simulink model "Controller_CS3"  (R2014a)
settings: Solver=ode4  StartTime=0.0  StopTime=Inf  FixedStep=0.01  MaxStep=0.01  RelTol=1e-3
undefined symbols (not defined in the file): Control, T_m_inv, T_matrix
libraries: simulink_extras x4, commnoisgen2 x1
(part 2 of 3)

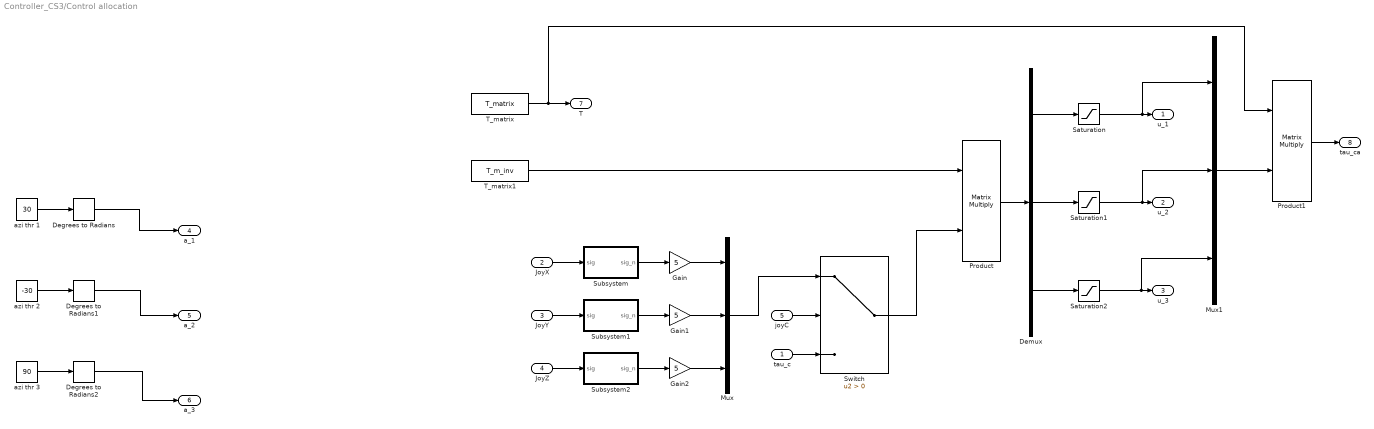
== system Controller_CS3/Control allocation ==
  tau_c : Inport  PortDimensions=3
  JoyX : Inport  Port=2  PortDimensions=1
  JoyY : Inport  Port=3  PortDimensions=1
  JoyZ : Inport  Port=4  PortDimensions=1
  joyC : Inport  Port=5  PortDimensions=1
  Degrees to Radians : simulink_extras/Transformations/Degrees to Radians
  Degrees to Radians1 : simulink_extras/Transformations/Degrees to Radians
  Degrees to Radians2 : simulink_extras/Transformations/Degrees to Radians
  Demux : Demux  Outputs=3
  Gain : Gain  Gain=5
  Gain1 : Gain  Gain=5
  Gain2 : Gain  Gain=5
  Mux : Mux  Inputs=3
  Mux1 : Mux  Inputs=3
  Product : Product  Multiplication=Matrix(*)
  Product1 : Product  Multiplication=Matrix(*)
  Saturation : Saturate  UpperLimit=13  LowerLimit=-13
  Saturation1 : Saturate  UpperLimit=13  LowerLimit=-13
  Saturation2 : Saturate  UpperLimit=8  LowerLimit=-8
  Subsystem : Subsystem
  Subsystem1 : Subsystem
  Subsystem2 : Subsystem
  Switch : Switch  Criteria=u2 > Threshold
  T_matrix : Constant  Value=T_matrix  VectorParams1D=off
  T_matrix1 : Constant  Value=T_m_inv  VectorParams1D=off
  azi thr 1 : Constant  Value=30
  azi thr 2 : Constant  Value=-30
  azi thr 3 : Constant  Value=90
  u_1 : Outport  PortDimensions=1
  u_2 : Outport  Port=2  PortDimensions=1
  u_3 : Outport  Port=3  PortDimensions=1
  a_1 : Outport  Port=4
  a_2 : Outport  Port=5
  a_3 : Outport  Port=6
  T : Outport  Port=7
  tau_ca : Outport  Port=8
  wires:
  azi thr 1/1 -> Degrees to Radians/1
  azi thr 2/1 -> Degrees to Radians1/1
  azi thr 3/1 -> Degrees to Radians2/1
  Degrees to Radians/1 -> a_1/1
  Degrees to Radians1/1 -> a_2/1
  Degrees to Radians2/1 -> a_3/1
  Product/1 -> Demux/1
  T_matrix1/1 -> Product/1
  JoyX/1 -> Subsystem/1(sig)
  JoyY/1 -> Subsystem1/1(sig)
  JoyZ/1 -> Subsystem2/1(sig)
  joyC/1 -> Switch/2
  Subsystem2/1(sig_n) -> Gain2/1
  Subsystem1/1(sig_n) -> Gain1/1
  Subsystem/1(sig_n) -> Gain/1
  Mux/1 -> Switch/1
  tau_c/1 -> Switch/3
  Switch/1 -> Product/2
  Gain/1 -> Mux/1
  Gain1/1 -> Mux/2
  Gain2/1 -> Mux/3
  Mux1/1 -> Product1/2
  T_matrix/1 -> Product1/1, T/1
  Product1/1 -> tau_ca/1
  Demux/3 -> Saturation2/1
  Demux/2 -> Saturation1/1
  Demux/1 -> Saturation/1
  Saturation1/1 -> Mux1/2, u_2/1
  Saturation2/1 -> Mux1/3, u_3/1
  Saturation/1 -> Mux1/1, u_1/1

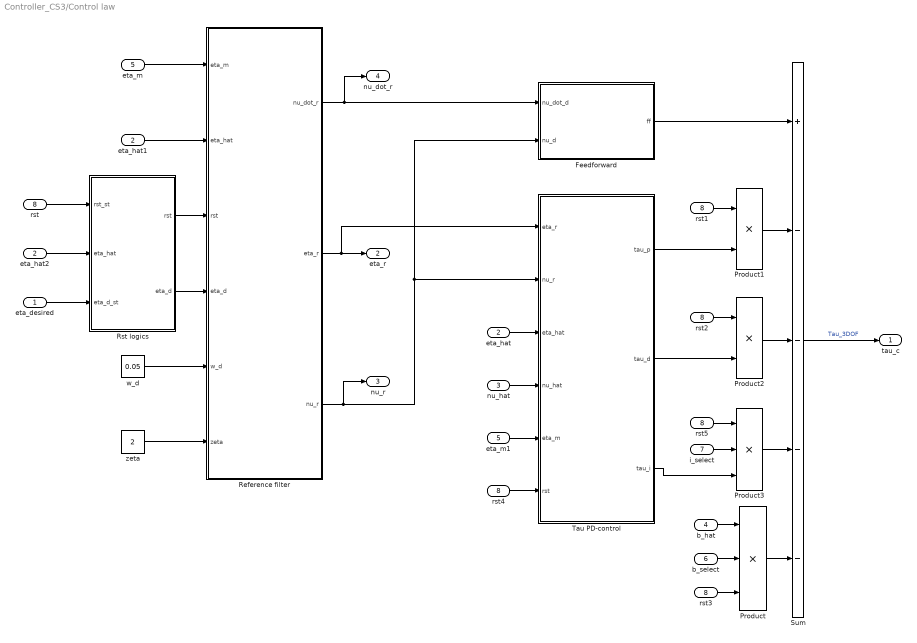
== system Controller_CS3/Control law ==
  eta_desired : Inport
  eta_hat : Inport  Port=2
  nu_hat : Inport  Port=3
  b_hat : Inport  Port=4
  eta_m : Inport  Port=5
  b_select : Inport  Port=6
  i_select : Inport  Port=7
  rst : Inport  Port=8
  Feedforward : Subsystem
  Product : Product  Inputs=3
  Product1 : Product
  Product2 : Product
  Product3 : Product  Inputs=3
  Reference filter : Subsystem
  Rst logics : Subsystem
  Sum : Sum  Inputs=+----  SaturateOnIntegerOverflow=on
  Tau PD-control : Subsystem
  eta_hat1 : InportShadow  Port=2
  eta_hat2 : InportShadow  Port=2
  eta_m1 : InportShadow  Port=5
  rst{1..5} (5 alike) : InportShadow  Port=8
  w_d : Constant  Value=0.05
  zeta : Constant  Value=2
  tau_c : Outport
  eta_r : Outport  Port=2
  nu_r : Outport  Port=3
  nu_dot_r : Outport  Port=4
  wires:
  Sum/1 -> tau_c/1  "Tau_3DOF"
  eta_hat/1 -> Tau PD-control/3(eta_hat)
  nu_hat/1 -> Tau PD-control/4(nu_hat)
  b_hat/1 -> Product/1
  Reference filter/1(nu_dot_r) -> nu_dot_r/1, Feedforward/1(nu_dot_d)
  Reference filter/2(eta_r) -> eta_r/1, Tau PD-control/1(eta_r)
  Reference filter/3(nu_r) -> Feedforward/2(nu_d), Tau PD-control/2(nu_r), nu_r/1
  eta_m1/1 -> Tau PD-control/5(eta_m)
  b_select/1 -> Product/2
  Rst logics/1(rst) -> Reference filter/3(rst)
  Rst logics/2(eta_d) -> Reference filter/4(eta_d)
  eta_m/1 -> Reference filter/1(eta_m)
  eta_desired/1 -> Rst logics/3(eta_d_st)
  rst/1 -> Rst logics/1(rst_st)
  eta_hat1/1 -> Reference filter/2(eta_hat)
  w_d/1 -> Reference filter/5(w_d)
  zeta/1 -> Reference filter/6(zeta)
  Product1/1 -> Sum/2
  rst1/1 -> Product1/1
  rst2/1 -> Product2/1
  rst3/1 -> Product/3
  eta_hat2/1 -> Rst logics/2(eta_hat)
  rst4/1 -> Tau PD-control/6(rst)
  Product/1 -> Sum/5
  Tau PD-control/3(tau_i) -> Product3/3
  rst5/1 -> Product3/1
  Feedforward/1(ff) -> Sum/1
  Product3/1 -> Sum/4
  Product2/1 -> Sum/3
  Tau PD-control/2(tau_d) -> Product2/2
  Tau PD-control/1(tau_p) -> Product1/2
  i_select/1 -> Product3/2

== system Controller_CS3/CyberShip3Model ==
  note: nu
  note: nu_dot
  note: etadot
  tau : Inport
  D : Gain  Gain=Control.VessObs.D  Multiplication=Matrix(K*u)  SaturateOnIntegerOverflow=on  OutDataTypeStr=Inherit: Same as input  ParamDataTypeStr=Inherit: Same as input
  Integrator1 : Integrator
  Integrator2 : Integrator
  Rotation matrix in yaw 1 : Subsystem  AncestorBlock=marine_gnc/Models/ Kinematics/Rotation matrix in yaw
      mask help:
      | b = R(psi)* a
      |
      | where
      |
      | input 1:    psi
      | input 2:    a - vector dim 3
      | output 1:  b - vector dim 3
      mask Display:
      | port_label('output', 1, 'R(psi)*v')
      | port_label('input', 1, 'psi')
      | port_label('input', 2, 'v')
  Sum3 : Sum  Inputs=+-  SaturateOnIntegerOverflow=on  InputSameDT=on  OutDataTypeStr=Inherit: Same as first input
  inv(M) : Gain  Gain=Control.VessObs.M_inv  Multiplication=Matrix(K*u)  SaturateOnIntegerOverflow=on  OutDataTypeStr=Inherit: Same as input  ParamDataTypeStr=Inherit: Same as input
  psi : Selector  InputPortWidth=3  Indices=[3]
  eta : Outport
  nu : Outport  Port=2
  wires:
  Integrator2/1 -> Rotation matrix in yaw 1/2(nu), nu/1, D/1
  D/1 -> Sum3/2
  Sum3/1 -> inv(M)/1
  inv(M)/1 -> Integrator2/1
  Rotation matrix in yaw 1/1(R*nu) -> Integrator1/1
  Integrator1/1 -> eta/1, psi/1
  psi/1 -> Rotation matrix in yaw 1/1(psi)
  tau/1 -> Sum3/1

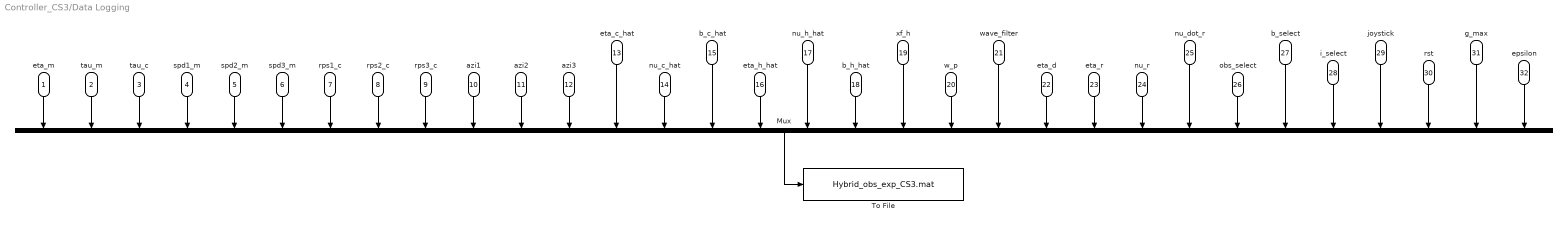
== system Controller_CS3/Data Logging ==
  eta_m : Inport
  tau_m : Inport  Port=2
  tau_c : Inport  Port=3
  spd1_m : Inport  Port=4
  spd2_m : Inport  Port=5
  spd3_m : Inport  Port=6
  rps1_c : Inport  Port=7
  rps2_c : Inport  Port=8
  rps3_c : Inport  Port=9
  azi1 : Inport  Port=10
  azi2 : Inport  Port=11
  azi3 : Inport  Port=12
  eta_c_hat : Inport  Port=13
  nu_c_hat : Inport  Port=14
  b_c_hat : Inport  Port=15
  eta_h_hat : Inport  Port=16
  nu_h_hat : Inport  Port=17
  b_h_hat : Inport  Port=18
  xf_h : Inport  Port=19
  w_p : Inport  Port=20
  wave_filter : Inport  Port=21
  eta_d : Inport  Port=22
  eta_r : Inport  Port=23
  nu_r : Inport  Port=24
  nu_dot_r : Inport  Port=25
  obs_select : Inport  Port=26
  b_select : Inport  Port=27
  i_select : Inport  Port=28
  joystick : Inport  Port=29
  rst : Inport  Port=30
  g_max : Inport  Port=31
  epsilon : Inport  Port=32
  Mux : Mux  Inputs=32
  To File : ToFile  Filename=Hybrid_obs_exp_CS3.mat  MatrixName=data  SampleTime=0.01
  wires:
  eta_m/1 -> Mux/1
  Mux/1 -> To File/1
  tau_m/1 -> Mux/2
  tau_c/1 -> Mux/3
  spd1_m/1 -> Mux/4
  spd2_m/1 -> Mux/5
  spd3_m/1 -> Mux/6
  rps1_c/1 -> Mux/7
  rps2_c/1 -> Mux/8
  rps3_c/1 -> Mux/9
  azi1/1 -> Mux/10
  azi2/1 -> Mux/11
  azi3/1 -> Mux/12
  eta_c_hat/1 -> Mux/13
  nu_c_hat/1 -> Mux/14
  b_c_hat/1 -> Mux/15
  eta_h_hat/1 -> Mux/16
  nu_h_hat/1 -> Mux/17
  b_h_hat/1 -> Mux/18
  xf_h/1 -> Mux/19
  w_p/1 -> Mux/20
  wave_filter/1 -> Mux/21
  eta_r/1 -> Mux/23
  eta_d/1 -> Mux/22
  nu_r/1 -> Mux/24
  obs_select/1 -> Mux/26
  nu_dot_r/1 -> Mux/25
  b_select/1 -> Mux/27
  i_select/1 -> Mux/28
  joystick/1 -> Mux/29
  rst/1 -> Mux/30
  g_max/1 -> Mux/31
  epsilon/1 -> Mux/32

== system Controller_CS3/Fake signal generator ==
  Gain : Gain  Gain=0.5
  Gain1 : Gain  Gain=diag([1 1 0.1])  Multiplication=Matrix(K*u)
  Gain2 : Gain  Gain=0
  Gaussian Noise Generator : commnoisgen2/Gaussian Noise Generator  m=[0 0 0]'  d=[1 1 0.25]'  s=[41 42 45]'  Ts=0.01  frameBased=off  sampPerFrame=1  orient=off  outDataType=double
  Integrator : Integrator
  Integrator1 : Integrator
  Integrator2 : Integrator
  Mux : Mux  Inputs=3
  Step : Step  Time=20  SampleTime=0
  Step1 : Step  Time=30  SampleTime=0
  Step2 : Step  Time=30  After=25*pi/180  SampleTime=0
  Sum : Sum  Inputs=|+-
  Sum1 : Sum  Inputs=|++
  Sum2 : Sum  Inputs=|+-
  eta_f : Outport
  wires:
  Gaussian Noise Generator/1 -> Integrator1/1
  Sum/1 -> Gain/1
  Gain/1 -> Integrator/1
  Integrator1/1 -> Sum/1
  Integrator/1 -> Sum1/1, Sum/2
  Sum1/1 -> Gain1/1
  Step/1 -> Mux/1
  Step1/1 -> Mux/2
  Step2/1 -> Mux/3
  Sum2/1 -> Gain2/1
  Integrator2/1 -> Sum1/2, Sum2/2
  Gain2/1 -> Integrator2/1
  Mux/1 -> Sum2/1
  Gain1/1 -> eta_f/1

== system Controller_CS3/Generalized force computation ==
  rps1 : Inport  PortDimensions=1
  rps2 : Inport  Port=2  PortDimensions=1
  rps3 : Inport  Port=3  PortDimensions=1
  T : Inport  Port=4
  Constant : Constant  Value=0.3507
  Constant1 : Constant  Value=0.2423
  Constant10 : Constant  Value=0.05
  Constant11 : Constant  Value=1024
  Constant2 : Constant  Value=0.09
  Constant3 : Constant  Value=1024
  Constant4 : Constant  Value=0.3464
  Constant5 : Constant  Value=0.2402
  Constant6 : Constant  Value=0.09
  Constant7 : Constant  Value=1024
  Constant8 : Constant  Value=0.1790
  Constant9 : Constant  Value=0.2383
  MATLAB Function : MATLAB Function  TreatAsAtomicUnit=on
  MATLAB Function1 : MATLAB Function  TreatAsAtomicUnit=on
  MATLAB Function2 : MATLAB Function  TreatAsAtomicUnit=on
  Mux : Mux  Inputs=3
  Product : Product  Multiplication=Matrix(*)
  tau_m : Outport
  wires:
  rps2/1 -> MATLAB Function1/1(rps)
  rps3/1 -> MATLAB Function2/1(rps)
  Mux/1 -> Product/2
  Product/1 -> tau_m/1
  T/1 -> Product/1
  Constant/1 -> MATLAB Function/2(Kt_p)
  Constant1/1 -> MATLAB Function/3(Kt_n)
  Constant2/1 -> MATLAB Function/4(d)
  Constant3/1 -> MATLAB Function/5(rho)
  rps1/1 -> MATLAB Function/1(rps)
  MATLAB Function/1(u) -> Mux/1
  Constant4/1 -> MATLAB Function1/2(Kt_p)
  Constant5/1 -> MATLAB Function1/3(Kt_n)
  Constant6/1 -> MATLAB Function1/4(d)
  Constant7/1 -> MATLAB Function1/5(rho)
  Constant8/1 -> MATLAB Function2/3(Kt_n)
  Constant10/1 -> MATLAB Function2/4(d)
  Constant9/1 -> MATLAB Function2/2(Kt_p)
  Constant11/1 -> MATLAB Function2/5(rho)
  MATLAB Function1/1(u) -> Mux/2
  MATLAB Function2/1(u) -> Mux/3

== system Controller_CS3/Norm ==
  m : Inport
  est : Inport  Port=2
  Demux : Demux  Outputs=3
  Math Function : Math  Operator=square  SaturateOnIntegerOverflow=on
  Math Function1 : Math  Operator=square  SaturateOnIntegerOverflow=on
  Math Function2 : Math  Operator=square  SaturateOnIntegerOverflow=on
  Sqrt : Sqrt  SaturateOnIntegerOverflow=on
  Sum : Sum  Inputs=+++
  Sum1 : Sum  Inputs=+-
  Out1 : Outport
  wires:
  Demux/1 -> Math Function/1
  Demux/2 -> Math Function1/1
  Demux/3 -> Math Function2/1
  Math Function1/1 -> Sum/2
  Math Function/1 -> Sum/1
  Math Function2/1 -> Sum/3
  Sum/1 -> Sqrt/1
  Sum1/1 -> Demux/1
  Sqrt/1 -> Out1/1
  est/1 -> Sum1/2
  m/1 -> Sum1/1

== system Controller_CS3/Norm1 ==
  m : Inport
  est : Inport  Port=2
  Demux : Demux  Outputs=3
  Math Function : Math  Operator=square  SaturateOnIntegerOverflow=on
  Math Function1 : Math  Operator=square  SaturateOnIntegerOverflow=on
  Math Function2 : Math  Operator=square  SaturateOnIntegerOverflow=on
  Sqrt : Sqrt  SaturateOnIntegerOverflow=on
  Sum : Sum  Inputs=+++
  Sum1 : Sum  Inputs=+-
  Out1 : Outport
  wires:
  m/1 -> Sum1/1
  est/1 -> Sum1/2
  Sqrt/1 -> Out1/1
  Sum1/1 -> Demux/1
  Sum/1 -> Sqrt/1
  Math Function2/1 -> Sum/3
  Math Function/1 -> Sum/1
  Math Function1/1 -> Sum/2
  Demux/3 -> Math Function2/1
  Demux/2 -> Math Function1/1
  Demux/1 -> Math Function/1

== system Controller_CS3/Observer selection logic ==
  eta_c_hat : Inport
  nu_c_hat : Inport  Port=2
  b_c_hat : Inport  Port=3
  eta_h_hat : Inport  Port=4
  nu_h_hat : Inport  Port=5
  b_h_hat : Inport  Port=6
  Observer_select : Inport  Port=7
  Mux : Mux  Inputs=3
  Mux1 : Mux  Inputs=3
  Switch1 : Switch  Criteria=u2 > Threshold
  b select : Selector  InputPortWidth=9  Indices=[7 8 9]
  eta select : Selector  InputPortWidth=9  Indices=[1 2 3]
  nu select : Selector  InputPortWidth=9  Indices=[4 5 6]
  eta_hat : Outport
  nu_hat : Outport  Port=2
  b_hat : Outport  Port=3
  wires:
  Mux/1 -> Switch1/1
  Mux1/1 -> Switch1/3
  Observer_select/1 -> Switch1/2
  eta_c_hat/1 -> Mux1/1
  nu_c_hat/1 -> Mux1/2
  b_c_hat/1 -> Mux1/3
  eta_h_hat/1 -> Mux/1
  nu_h_hat/1 -> Mux/2
  b_h_hat/1 -> Mux/3
  eta select/1 -> eta_hat/1
  Switch1/1 -> eta select/1, b select/1, nu select/1
  nu select/1 -> nu_hat/1
  b select/1 -> b_hat/1

== system Controller_CS3/Observers ==
  eta_m : Inport
  tau_m : Inport  Port=2
  w_p : Inport  Port=3
  wave_filter : Inport  Port=4
  g_max : Inport  Port=5
  epsilon : Inport  Port=6
  Cont. Nonlinear Passive DP obs : Subsystem
  Hybrid Nonlinear Passive DP obs : Subsystem
  eta_m1 : InportShadow
  tau_m1 : InportShadow  Port=2
  eta_c_hat : Outport
  nu_c_hat : Outport  Port=2
  b_c_hat : Outport  Port=3
  eta_h_hat : Outport  Port=4
  nu_h_hat : Outport  Port=5
  b_h_hat : Outport  Port=6
  xf_h : Outport  Port=7
  wires:
  eta_m/1 -> Cont. Nonlinear Passive DP obs/1(eta_m)
  Cont. Nonlinear Passive DP obs/1(eta_hat) -> eta_c_hat/1
  Cont. Nonlinear Passive DP obs/2(nu_hat) -> nu_c_hat/1
  Cont. Nonlinear Passive DP obs/3(b_hat) -> b_c_hat/1
  tau_m/1 -> Cont. Nonlinear Passive DP obs/2(tau_c)
  Hybrid Nonlinear Passive DP obs/1(eta_hat) -> eta_h_hat/1
  Hybrid Nonlinear Passive DP obs/2(nu_hat) -> nu_h_hat/1
  Hybrid Nonlinear Passive DP obs/3(b_hat) -> b_h_hat/1
  tau_m1/1 -> Hybrid Nonlinear Passive DP obs/2(tau)
  eta_m1/1 -> Hybrid Nonlinear Passive DP obs/1(eta_m)
  wave_filter/1 -> Hybrid Nonlinear Passive DP obs/4(wave_filter), Cont. Nonlinear Passive DP obs/4(wave_filter)
  Hybrid Nonlinear Passive DP obs/4(xf_h) -> xf_h/1
  epsilon/1 -> Hybrid Nonlinear Passive DP obs/6(epsilon)
  g_max/1 -> Hybrid Nonlinear Passive DP obs/5(g_max)
  w_p/1 -> Hybrid Nonlinear Passive DP obs/3(w_p), Cont. Nonlinear Passive DP obs/3(w_p)

== system Controller_CS3/Subsystem ==
  In1 : Inport
  Degrees to Radians : simulink_extras/Transformations/Degrees to Radians
  Demux : Demux  Outputs=3
  Gain : Gain  Gain=1/1000
  Gain1 : Gain  Gain=1/1000
  Mux : Mux  Inputs=3
  Out1 : Outport
  wires:
  In1/1 -> Demux/1
  Mux/1 -> Out1/1
  Demux/3 -> Degrees to Radians/1
  Degrees to Radians/1 -> Mux/3
  Demux/2 -> Gain/1
  Demux/1 -> Gain1/1
  Gain/1 -> Mux/2
  Gain1/1 -> Mux/1

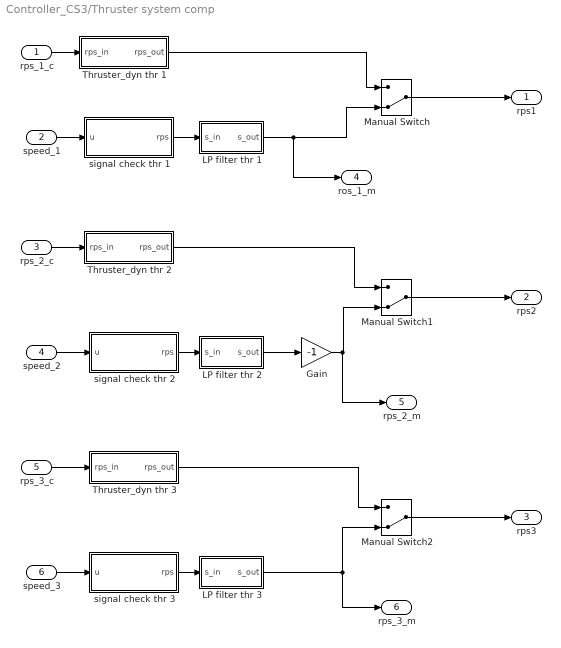
== system Controller_CS3/Thruster system comp ==
  rps_1_c : Inport
  speed_1 : Inport  Port=2
  rps_2_c : Inport  Port=3
  speed_2 : Inport  Port=4
  rps_3_c : Inport  Port=5
  speed_3 : Inport  Port=6
  Gain : Gain  Gain=-1
  LP filter thr 1 : Subsystem
  LP filter thr 2 : Subsystem
  LP filter thr 3 : Subsystem
  Manual Switch : ManualSwitch  CurrentSetting=0
  Manual Switch1 : ManualSwitch  CurrentSetting=0
  Manual Switch2 : ManualSwitch  CurrentSetting=0
  Thruster_dyn thr 1 : Subsystem
  Thruster_dyn thr 2 : Subsystem
  Thruster_dyn thr 3 : Subsystem
  signal check thr 1 : MATLAB Function  TreatAsAtomicUnit=on
  signal check thr 2 : MATLAB Function  TreatAsAtomicUnit=on
  signal check thr 3 : MATLAB Function  TreatAsAtomicUnit=on
  rps1 : Outport
  rps2 : Outport  Port=2
  rps3 : Outport  Port=3
  ros_1_m : Outport  Port=4
  rps_2_m : Outport  Port=5
  rps_3_m : Outport  Port=6
  wires:
  Manual Switch/1 -> rps1/1
  Manual Switch2/1 -> rps3/1
  Manual Switch1/1 -> rps2/1
  rps_1_c/1 -> Thruster_dyn thr 1/1(rps_in)
  Thruster_dyn thr 1/1(rps_out) -> Manual Switch/1
  Thruster_dyn thr 2/1(rps_out) -> Manual Switch1/1
  signal check thr 1/1(rps) -> LP filter thr 1/1(s_in)
  signal check thr 2/1(rps) -> LP filter thr 2/1(s_in)
  signal check thr 3/1(rps) -> LP filter thr 3/1(s_in)
  speed_2/1 -> signal check thr 2/1(u)
  speed_3/1 -> signal check thr 3/1(u)
  speed_1/1 -> signal check thr 1/1(u)
  LP filter thr 1/1(s_out) -> Manual Switch/2, ros_1_m/1
  LP filter thr 2/1(s_out) -> Gain/1
  rps_2_c/1 -> Thruster_dyn thr 2/1(rps_in)
  rps_3_c/1 -> Thruster_dyn thr 3/1(rps_in)
  Thruster_dyn thr 3/1(rps_out) -> Manual Switch2/1
  Gain/1 -> rps_2_m/1, Manual Switch1/2
  LP filter thr 3/1(s_out) -> rps_3_m/1, Manual Switch2/2

== system Controller_CS3/u 2 rps ==
  u : Inport
  Constant : Constant  Value=0.3507
  Constant1 : Constant  Value=0.2423
  Constant2 : Constant  Value=0.09
  Constant3 : Constant  Value=1024
  MATLAB Function : MATLAB Function  TreatAsAtomicUnit=on
  rps : Outport
  wires:
  u/1 -> MATLAB Function/1(u)
  MATLAB Function/1(rps) -> rps/1
  Constant/1 -> MATLAB Function/2(Kt_p)
  Constant1/1 -> MATLAB Function/3(Kt_n)
  Constant2/1 -> MATLAB Function/4(d)
  Constant3/1 -> MATLAB Function/5(rho)

== system Controller_CS3/u 2 rps1 ==
  u : Inport
  Constant : Constant  Value=0.3464
  Constant1 : Constant  Value=0.2402
  Constant2 : Constant  Value=0.09
  Constant3 : Constant  Value=1024
  MATLAB Function : MATLAB Function  TreatAsAtomicUnit=on
  rps : Outport
  wires:
  Constant3/1 -> MATLAB Function/5(rho)
  Constant2/1 -> MATLAB Function/4(d)
  Constant1/1 -> MATLAB Function/3(Kt_n)
  Constant/1 -> MATLAB Function/2(Kt_p)
  MATLAB Function/1(rps) -> rps/1
  u/1 -> MATLAB Function/1(u)

== system Controller_CS3/u 2 rps2 ==
  u : Inport
  Constant : Constant  Value=0.1790
  Constant1 : Constant  Value=0.2383
  Constant2 : Constant  Value=0.05
  Constant3 : Constant  Value=1024
  MATLAB Function : MATLAB Function  TreatAsAtomicUnit=on
  rps : Outport
  wires:
  u/1 -> MATLAB Function/1(u)
  MATLAB Function/1(rps) -> rps/1
  Constant2/1 -> MATLAB Function/4(d)
  Constant3/1 -> MATLAB Function/5(rho)
  Constant/1 -> MATLAB Function/3(Kt_n)
  Constant1/1 -> MATLAB Function/2(Kt_p)

== system Controller_CS3/Control allocation/Subsystem ==
  sig : Inport
  Constant : Constant  Value=2^15
  Divide : Product  Inputs=*/
  sig_n : Outport
  wires:
  sig/1 -> Divide/1
  Constant/1 -> Divide/2
  Divide/1 -> sig_n/1

== system Controller_CS3/Control allocation/Subsystem1 ==
  sig : Inport
  Constant : Constant  Value=2^15
  Divide : Product  Inputs=*/
  sig_n : Outport
  wires:
  Divide/1 -> sig_n/1
  Constant/1 -> Divide/2
  sig/1 -> Divide/1

== system Controller_CS3/Control allocation/Subsystem2 ==
  sig : Inport
  Constant : Constant  Value=2^15
  Divide : Product  Inputs=*/
  sig_n : Outport
  wires:
  sig/1 -> Divide/1
  Constant/1 -> Divide/2
  Divide/1 -> sig_n/1

== system Controller_CS3/Control law/Feedforward ==
  nu_dot_d : Inport
  nu_d : Inport  Port=2
  Gain : Gain  Gain=Control.Vessel_3_DOF.M  Multiplication=Matrix(K*u)  SaturateOnIntegerOverflow=on  OutDataTypeStr=Inherit: Same as input  ParamDataTypeStr=Inherit: Same as input
  Gain1 : Gain  Gain=Control.Vessel_3_DOF.D  Multiplication=Matrix(K*u)  SaturateOnIntegerOverflow=on  OutDataTypeStr=Inherit: Same as input  ParamDataTypeStr=Inherit: Same as input
  Sum : Sum  Inputs=+|+  SaturateOnIntegerOverflow=on
  ff : Outport
  wires:
  nu_d/1 -> Gain1/1
  nu_dot_d/1 -> Gain/1
  Gain/1 -> Sum/2
  Sum/1 -> ff/1
  Gain1/1 -> Sum/1

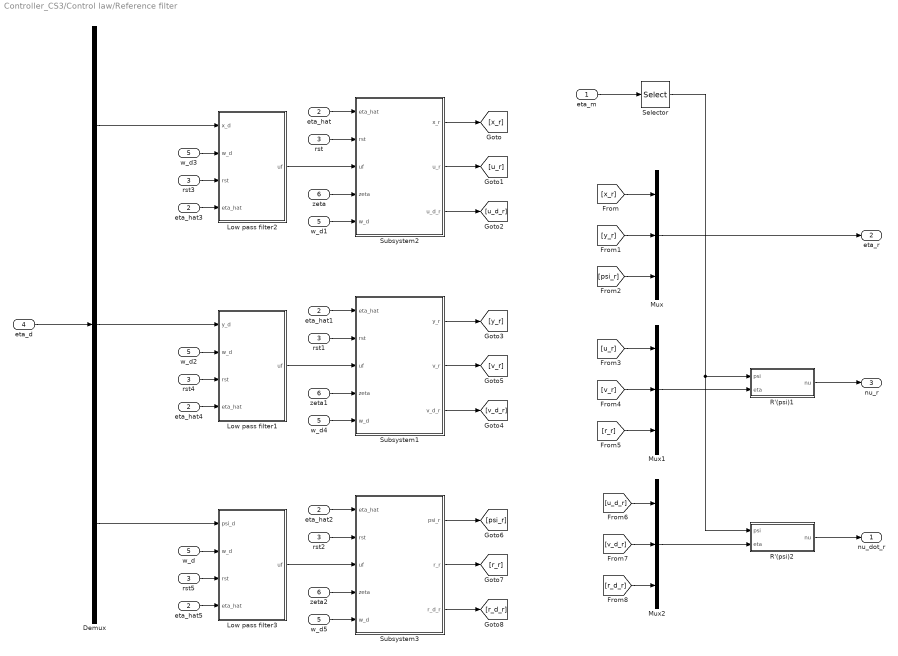
== system Controller_CS3/Control law/Reference filter ==
  eta_m : Inport
  eta_hat : Inport  Port=2
  rst : Inport  Port=3
  eta_d : Inport  Port=4
  w_d : Inport  Port=5
  zeta : Inport  Port=6
  Demux : Demux  Outputs=3
  Low pass filter1 : Subsystem
  Low pass filter2 : Subsystem
  Low pass filter3 : Subsystem
  Mux : Mux  Inputs=3
  Mux1 : Mux  Inputs=3
  Mux2 : Mux  Inputs=3
  R'(psi)1 : Subsystem
  R'(psi)2 : Subsystem
  Selector : Selector  InputPortWidth=3  Indices=[3]
  Subsystem1 : Subsystem
  Subsystem2 : Subsystem
  Subsystem3 : Subsystem
  eta_hat{1..5} (5 alike) : InportShadow  Port=2
  rst{1..5} (5 alike) : InportShadow  Port=3
  w_d{1..5} (5 alike) : InportShadow  Port=5
  zeta1 : InportShadow  Port=6
  zeta2 : InportShadow  Port=6
  nu_dot_r : Outport  PortDimensions=3
  eta_r : Outport  Port=2  PortDimensions=3
  nu_r : Outport  Port=3  PortDimensions=3
  wires:
  eta_d/1 -> Demux/1
  Demux/3 -> Low pass filter3/1(psi_d)
  w_d/1 -> Low pass filter3/2(w_d)
  Demux/1 -> Low pass filter2/1(x_d)
  w_d3/1 -> Low pass filter2/2(w_d)
  Mux1/1 -> R'(psi)1/2(eta)
  Mux2/1 -> R'(psi)2/2(eta)
  Mux/1 -> eta_r/1
  R'(psi)1/1(nu) -> nu_r/1
  R'(psi)2/1(nu) -> nu_dot_r/1
  eta_m/1 -> Selector/1
  Selector/1 -> R'(psi)2/1(psi), R'(psi)1/1(psi)
  zeta/1 -> Subsystem2/4(zeta)
  rst/1 -> Subsystem2/2(rst)
  eta_hat1/1 -> Subsystem1/1(eta_hat)
  rst1/1 -> Subsystem1/2(rst)
  zeta1/1 -> Subsystem1/4(zeta)
  Subsystem2/1(x_r) -> [x_r]
  Subsystem2/2(u_r) -> [u_r]
  Subsystem2/3(u_d_r) -> [u_d_r]
  Subsystem1/1(y_r) -> [y_r]
  Subsystem1/2(v_r) -> [v_r]
  Subsystem1/3(v_d_r) -> [v_d_r]
  [x_r] -> Mux/1
  [psi_r] -> Mux/3
  [y_r] -> Mux/2
  [r_r] -> Mux1/3
  [v_r] -> Mux1/2
  [u_r] -> Mux1/1
  [r_d_r] -> Mux2/3
  [v_d_r] -> Mux2/2
  [u_d_r] -> Mux2/1
  Low pass filter2/1(uf) -> Subsystem2/3(uf)
  rst3/1 -> Low pass filter2/3(rst)
  eta_hat/1 -> Subsystem2/1(eta_hat)
  eta_hat3/1 -> Low pass filter2/4(eta_hat)
  w_d1/1 -> Subsystem2/5(w_d)
  Demux/2 -> Low pass filter1/1(y_d)
  w_d2/1 -> Low pass filter1/2(w_d)
  rst4/1 -> Low pass filter1/3(rst)
  eta_hat4/1 -> Low pass filter1/4(eta_hat)
  Low pass filter1/1(uf) -> Subsystem1/3(uf)
  w_d4/1 -> Subsystem1/5(w_d)
  rst5/1 -> Low pass filter3/3(rst)
  eta_hat5/1 -> Low pass filter3/4(eta_hat)
  eta_hat2/1 -> Subsystem3/1(eta_hat)
  rst2/1 -> Subsystem3/2(rst)
  Low pass filter3/1(uf) -> Subsystem3/3(uf)
  zeta2/1 -> Subsystem3/4(zeta)
  w_d5/1 -> Subsystem3/5(w_d)
  Subsystem3/1(psi_r) -> [psi_r]
  Subsystem3/2(r_r) -> [r_r]
  Subsystem3/3(r_d_r) -> [r_d_r]

== system Controller_CS3/Control law/Rst logics ==
  rst_st : Inport
  eta_hat : Inport  Port=2
  eta_d_st : Inport  Port=3
  MATLAB Function : MATLAB Function  TreatAsAtomicUnit=on
  Memory : Memory
  rst : Outport  PortDimensions=1
  eta_d : Outport  Port=2  PortDimensions=3
  wires:
  MATLAB Function/1(rst) -> rst/1
  MATLAB Function/2(eta_d) -> eta_d/1
  eta_d_st/1 -> Memory/1, MATLAB Function/3(eta_d_in)
  rst_st/1 -> MATLAB Function/1(rst_in)
  Memory/1 -> MATLAB Function/4(eta_d_prev)
  eta_hat/1 -> MATLAB Function/2(eta_hat)

== system Controller_CS3/Control law/Tau PD-control ==
  note: PD-control term in controller
  eta_r : Inport
  nu_r : Inport  Port=2
  eta_hat : Inport  Port=3
  nu_hat : Inport  Port=4
  eta_m : Inport  Port=5
  rst : Inport  Port=6
  Constant : Constant  Value=diag(Control.PID.Kp)
  Constant1 : Constant  Value=diag(Control.PID.Kd)
  Constant2 : Constant  Value=diag(Control.PID.Ki)
  "GNC: \"Transposed rotation matrix yaw: RTz_psi\"" : Subsystem
  Integrator : Integrator  ExternalReset=rising  LimitOutput=on  UpperSaturationLimit=inv(diag(Control.PID.Ki))*[4 4 4]'  LowerSaturationLimit=-inv(diag(Control.PID.Ki))*[4 4 4]'
  Product : Product  Multiplication=Matrix(*)
  Product1 : Product  Multiplication=Matrix(*)
  Product2 : Product  Multiplication=Matrix(*)
  Scope7 : Scope
      settings: YMin=-0.012  YMax=0.009  SaveName=ScopeData27
  Selector2 : Selector  InputPortWidth=3  Indices=[3]
  Sum : Sum  Inputs=+-|  SaturateOnIntegerOverflow=on
  Sum1 : Sum  Inputs=+-|  SaturateOnIntegerOverflow=on
  tau_p : Outport  PortDimensions=3
  tau_d : Outport  Port=2  PortDimensions=3
  tau_i : Outport  Port=3  PortDimensions=3
  wires:
  eta_hat/1 -> Sum/1
  nu_hat/1 -> Sum1/1
  Sum1/1 -> Product1/2
  Selector2/1 -> "GNC: \"Transposed rotation matrix yaw: RTz_psi\""/1(psi)
  "GNC: \"Transposed rotation matrix yaw: RTz_psi\""/1(R_T*nu) -> Integrator/1, Product/2
  nu_r/1 -> Sum1/2
  eta_r/1 -> Sum/2
  Product/1 -> tau_p/1
  eta_m/1 -> Selector2/1
  Constant/1 -> Product/1
  Product1/1 -> tau_d/1
  Constant1/1 -> Product1/1
  rst/1 -> Integrator/2
  Integrator/1 -> Product2/2
  Product2/1 -> tau_i/1
  Constant2/1 -> Product2/1
  Sum/1 -> Scope7/1, "GNC: \"Transposed rotation matrix yaw: RTz_psi\""/2(nu)

== system Controller_CS3/CyberShip3Model/Rotation matrix in yaw 1 ==
  psi : Inport
  nu : Inport  Port=2
  Fcn : Fcn  Expr=cos(u(1))*u(2)-sin(u(1))*u(3)
  Fcn1 : Fcn  Expr=sin(u(1))*u(2)+cos(u(1))*u(3)
  Fcn2 : Fcn  Expr=u(4)
  Mux : Mux  Inputs=2
  Mux1 : Mux  Inputs=3
  R*nu : Outport
  wires:
  nu/1 -> Mux/2
  psi/1 -> Mux/1
  Mux1/1 -> R*nu/1  "eta_dot"
  Fcn2/1 -> Mux1/3  "psi_dot"
  Fcn1/1 -> Mux1/2  "y_dot"
  Fcn/1 -> Mux1/1  "x_dot"
  Mux/1 -> Fcn/1, Fcn1/1, Fcn2/1

== system Controller_CS3/Observers/Cont. Nonlinear Passive DP obs ==
  eta_m : Inport
  tau_c : Inport  Port=2
  w_p : Inport  Port=3
  wave_filter : Inport  Port=4  PortDimensions=1
  Calc observer gains1 : Subsystem  mask{lmb=Control.VessObs.lmb{2}, k=Control.VessObs.k{2}, zeta=Control.VessObs.damp{2}, K3=Control.VessObs.K3{2}, K4=Control.VessObs.K4{2}}
      mask prompts: lmb "Control.VessObs.lmb{i}=lmb"; k "Control.VessObs.k{i}=k"; zeta "Control.VessObs.damp{i}=zeta"; K3 "Control.VessObs.K3{1}=K3"; K4 "Control.VessObs.K4{1}=K4"
  Nonlinear observer : Subsystem
  eta_hat : Outport
  nu_hat : Outport  Port=2
  b_hat : Outport  Port=3
  wires:
  Calc observer gains1/4(K3) -> Nonlinear observer/6(K3)
  Calc observer gains1/5(K5) -> Nonlinear observer/7(K5)
  Calc observer gains1/3(Aw(w_p)) -> Nonlinear observer/5(Aw)
  Calc observer gains1/2(K2(w_1)) -> Nonlinear observer/4(K2)
  Calc observer gains1/1(K1(w_p)) -> Nonlinear observer/3(K1)
  tau_c/1 -> Nonlinear observer/2(Tau)
  eta_m/1 -> Nonlinear observer/1(Eta_meas)
  Nonlinear observer/2(Nu_hat) -> nu_hat/1
  Nonlinear observer/1(Eta_hat) -> eta_hat/1
  Nonlinear observer/3(b_hat) -> b_hat/1
  w_p/1 -> Calc observer gains1/1(w_p)
  wave_filter/1 -> Nonlinear observer/8(Sim Wavefilter)

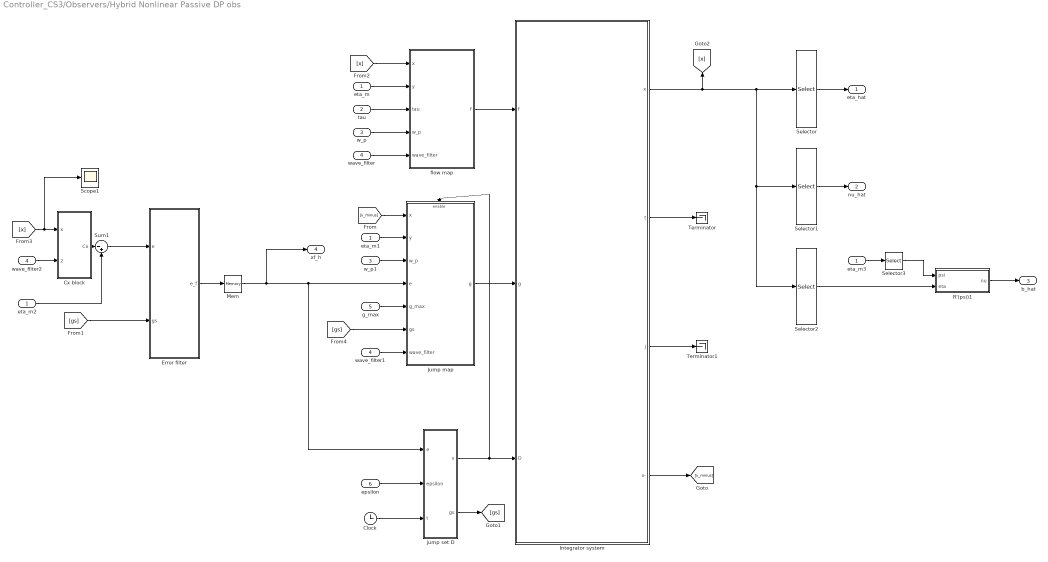
== system Controller_CS3/Observers/Hybrid Nonlinear Passive DP obs ==
  eta_m : Inport  PortDimensions=3
  tau : Inport  Port=2
  w_p : Inport  Port=3
  wave_filter : Inport  Port=4  PortDimensions=1
  g_max : Inport  Port=5  PortDimensions=3
  epsilon : Inport  Port=6  PortDimensions=3
  Clock : Clock
  Cx block : Subsystem
  Error filter : Subsystem
  Integrator system : Subsystem
  Jump map : Subsystem
  Mem : Memory
  R'(psi)1 : Subsystem
  Scope1 : Scope
      settings: SaveName=ScopeData2
  Selector : Selector  InputPortWidth=15  Indices=[7 8 9]
  Selector1 : Selector  InputPortWidth=15  Indices=[10 11 12]
  Selector2 : Selector  InputPortWidth=15  Indices=[13 14 15]
  Selector3 : Selector  InputPortWidth=3  Indices=3
  Sum1 : Sum  Inputs=|-+
  Terminator : Terminator
  Terminator1 : Terminator
  eta_m1 : InportShadow  PortDimensions=3
  eta_m2 : InportShadow  PortDimensions=3
  eta_m3 : InportShadow  PortDimensions=3
  flow map : Subsystem
  jump set D : MATLAB Function  TreatAsAtomicUnit=on
  w_p1 : InportShadow  Port=3
  wave_filter1 : InportShadow  Port=4  PortDimensions=1
  wave_filter2 : InportShadow  Port=4  PortDimensions=1
  eta_hat : Outport
  nu_hat : Outport  Port=2
  b_hat : Outport  Port=3
  xf_h : Outport  Port=4
  wires:
  Integrator system/1(x) -> [x], Selector2/1, Selector1/1, Selector/1
  Selector/1 -> eta_hat/1
  Selector1/1 -> nu_hat/1
  Integrator system/2(t) -> Terminator/1
  Integrator system/3(j) -> Terminator1/1
  flow map/1(f) -> Integrator system/1(f)
  eta_m/1 -> flow map/2(y)
  tau/1 -> flow map/3(tau)
  w_p/1 -> flow map/4(w_p)
  Clock/1 -> jump set D/3(t)
  Jump map/1(g) -> Integrator system/2(g)
  eta_m1/1 -> Jump map/2(y)
  w_p1/1 -> Jump map/3(w_p)
  Cx block/1(Cx) -> Sum1/1
  eta_m2/1 -> Sum1/2
  Integrator system/4(x-) -> [x_minus]
  [x_minus] -> Jump map/1(x)
  jump set D/2(gs) -> [gs]
  [x] -> flow map/1(x)
  Error filter/1(e_f) -> Mem/1
  wave_filter/1 -> flow map/5(wave_filter)
  wave_filter1/1 -> Jump map/7(wave_filter)
  [x] -> Scope1/1, Cx block/1(x)
  wave_filter2/1 -> Cx block/2(wave_filter)
  Sum1/1 -> Error filter/1(e)
  [gs] -> Error filter/2(gs)
  [gs] -> Jump map/6(gs)
  jump set D/1(v) -> Integrator system/3(D), Jump map/Enable
  Mem/1 -> xf_h/1, jump set D/1(e), Jump map/4(e)
  Selector2/1 -> R'(psi)1/2(eta)
  R'(psi)1/1(nu) -> b_hat/1
  eta_m3/1 -> Selector3/1
  Selector3/1 -> R'(psi)1/1(psi)
  g_max/1 -> Jump map/5(g_max)
  epsilon/1 -> jump set D/2(epsilon)

== system Controller_CS3/Thruster system comp/LP filter thr 1 ==
  s_in : Inport
  Gain : Gain  Gain=5
  Integrator : Integrator
  Sum : Sum  Inputs=|+-
  s_out : Outport
  wires:
  s_in/1 -> Sum/1
  Sum/1 -> Gain/1
  Gain/1 -> Integrator/1
  Integrator/1 -> s_out/1, Sum/2

== system Controller_CS3/Thruster system comp/LP filter thr 2 ==
  s_in : Inport
  Gain : Gain  Gain=5
  Integrator : Integrator
  Sum : Sum  Inputs=|+-
  s_out : Outport
  wires:
  Integrator/1 -> Sum/2, s_out/1
  Gain/1 -> Integrator/1
  Sum/1 -> Gain/1
  s_in/1 -> Sum/1

== system Controller_CS3/Thruster system comp/LP filter thr 3 ==
  s_in : Inport
  Gain : Gain  Gain=5
  Integrator : Integrator
  Sum : Sum  Inputs=|+-
  s_out : Outport
  wires:
  s_in/1 -> Sum/1
  Sum/1 -> Gain/1
  Gain/1 -> Integrator/1
  Integrator/1 -> s_out/1, Sum/2

== system Controller_CS3/Thruster system comp/Thruster_dyn thr 1 ==
  rps_in : Inport
  Gain : Gain  Gain=1/2.5
  Integrator : Integrator
  Sum : Sum  Inputs=|+-
  rps_out : Outport
  wires:
  Integrator/1 -> Sum/2, rps_out/1
  Gain/1 -> Integrator/1
  Sum/1 -> Gain/1
  rps_in/1 -> Sum/1

== system Controller_CS3/Thruster system comp/Thruster_dyn thr 2 ==
  rps_in : Inport
  Gain : Gain  Gain=1/2.5
  Integrator : Integrator
  Sum : Sum  Inputs=|+-
  rps_out : Outport
  wires:
  rps_in/1 -> Sum/1
  Sum/1 -> Gain/1
  Gain/1 -> Integrator/1
  Integrator/1 -> rps_out/1, Sum/2

== system Controller_CS3/Thruster system comp/Thruster_dyn thr 3 ==
  rps_in : Inport
  Gain : Gain  Gain=1/2.5
  Integrator : Integrator
  Sum : Sum  Inputs=|+-
  rps_out : Outport
  wires:
  Integrator/1 -> Sum/2, rps_out/1
  Gain/1 -> Integrator/1
  Sum/1 -> Gain/1
  rps_in/1 -> Sum/1

== system Controller_CS3/Control law/Reference filter/Low pass filter1 ==
  y_d : Inport
  w_d : Inport  Port=2
  rst : Inport  Port=3
  eta_hat : Inport  Port=4
  Integrator : Integrator  ExternalReset=rising  InitialConditionSource=external
  Product : Product  Inputs=4
  Product1 : Product
  Product2 : Product  Inputs=3
  Selector : Selector  InputPortWidth=3  Indices=[2]
  Sum : Sum  Inputs=|+-
  w_d1 : InportShadow  Port=2
  uf : Outport
  wires:
  Selector/1 -> Product2/1
  eta_hat/1 -> Selector/1
  Product2/1 -> Integrator/3
  w_d1/1 -> Product2/2, Product2/3
  rst/1 -> Integrator/2
  w_d/1 -> Product1/1, Product/2, Product/3, Product/1
  Product1/1 -> Sum/2
  Product/1 -> Sum/1
  y_d/1 -> Product/4
  Integrator/1 -> uf/1, Product1/2
  Sum/1 -> Integrator/1

== system Controller_CS3/Control law/Reference filter/Low pass filter2 ==
  x_d : Inport
  w_d : Inport  Port=2
  rst : Inport  Port=3
  eta_hat : Inport  Port=4
  Integrator : Integrator  ExternalReset=rising  InitialConditionSource=external
  Product : Product  Inputs=4
  Product1 : Product
  Product2 : Product  Inputs=3
  Selector : Selector  InputPortWidth=3  Indices=[1]
  Sum : Sum  Inputs=|+-
  w_d1 : InportShadow  Port=2
  uf : Outport
  wires:
  Sum/1 -> Integrator/1
  Integrator/1 -> Product1/2, uf/1
  x_d/1 -> Product/4
  Product/1 -> Sum/1
  Product1/1 -> Sum/2
  w_d/1 -> Product/1, Product/3, Product/2, Product1/1
  rst/1 -> Integrator/2
  w_d1/1 -> Product2/3, Product2/2
  Product2/1 -> Integrator/3
  eta_hat/1 -> Selector/1
  Selector/1 -> Product2/1

== system Controller_CS3/Control law/Reference filter/Low pass filter3 ==
  psi_d : Inport
  w_d : Inport  Port=2
  rst : Inport  Port=3
  eta_hat : Inport  Port=4
  Integrator : Integrator  ExternalReset=rising  InitialConditionSource=external
  Product : Product  Inputs=4
  Product1 : Product
  Product2 : Product  Inputs=3
  Selector : Selector  InputPortWidth=3  Indices=3
  Sum : Sum  Inputs=|+-
  w_d1 : InportShadow  Port=2
  uf : Outport
  wires:
  Sum/1 -> Integrator/1
  Integrator/1 -> Product1/2, uf/1
  psi_d/1 -> Product/4
  Product/1 -> Sum/1
  Product1/1 -> Sum/2
  w_d/1 -> Product/1, Product/3, Product/2, Product1/1
  rst/1 -> Integrator/2
  w_d1/1 -> Product2/3, Product2/2
  Product2/1 -> Integrator/3
  eta_hat/1 -> Selector/1
  Selector/1 -> Product2/1

== system Controller_CS3/Control law/Reference filter/R'(psi)1 ==
  psi : Inport
  eta : Inport  Port=2
  Demux : Demux  Outputs=3
  Mux : Mux  Inputs=3
  Mux1 : Mux  Inputs=3
  Row1 : Fcn  Expr=cos(u(3))*u(1)+sin(u(3))*u(2)
  Row2 : Fcn  Expr=-sin(u(3))*u(1)+cos(u(3))*u(2)
  nu : Outport
  wires:
  Row1/1 -> Mux1/1
  Row2/1 -> Mux1/2
  Mux1/1 -> nu/1
  Mux/1 -> Row2/1, Row1/1
  eta/1 -> Demux/1
  psi/1 -> Mux/3
  Demux/1 -> Mux/1
  Demux/2 -> Mux/2
  Demux/3 -> Mux1/3

== system Controller_CS3/Control law/Reference filter/R'(psi)2 ==
  psi : Inport
  eta : Inport  Port=2
  Demux : Demux  Outputs=3
  Mux : Mux  Inputs=3
  Mux1 : Mux  Inputs=3
  Row1 : Fcn  Expr=cos(u(3))*u(1)+sin(u(3))*u(2)
  Row2 : Fcn  Expr=-sin(u(3))*u(1)+cos(u(3))*u(2)
  nu : Outport
  wires:
  Demux/3 -> Mux1/3
  Demux/2 -> Mux/2
  Demux/1 -> Mux/1
  psi/1 -> Mux/3
  eta/1 -> Demux/1
  Mux/1 -> Row1/1, Row2/1
  Mux1/1 -> nu/1
  Row2/1 -> Mux1/2
  Row1/1 -> Mux1/1

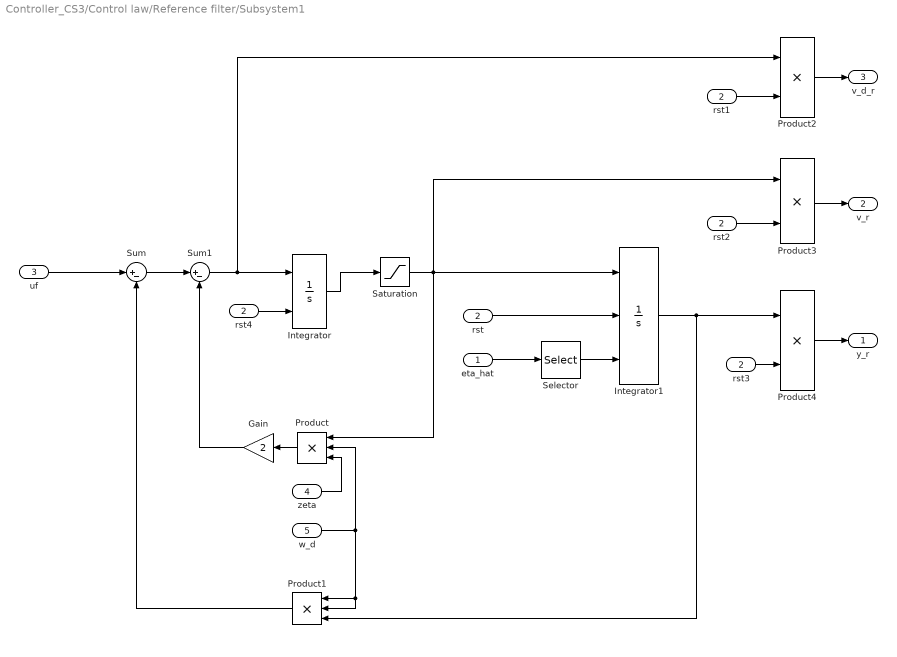
== system Controller_CS3/Control law/Reference filter/Subsystem1 ==
  eta_hat : Inport
  rst : Inport  Port=2
  uf : Inport  Port=3
  zeta : Inport  Port=4
  w_d : Inport  Port=5
  Gain : Gain  Gain=2
  Integrator : Integrator  ExternalReset=rising
  Integrator1 : Integrator  ExternalReset=either  InitialConditionSource=external
  Product : Product  Inputs=3
  Product1 : Product  Inputs=3
  Product2 : Product
  Product3 : Product
  Product4 : Product
  Saturation : Saturate  UpperLimit=0.05  LowerLimit=-0.05
  Selector : Selector  InputPortWidth=3  Indices=2
  Sum : Sum  Inputs=|+-
  Sum1 : Sum  Inputs=|+-
  rst{1..4} (4 alike) : InportShadow  Port=2
  y_r : Outport
  v_r : Outport  Port=2
  v_d_r : Outport  Port=3
  wires:
  rst4/1 -> Integrator/2
  rst3/1 -> Product4/2
  rst2/1 -> Product3/2
  rst1/1 -> Product2/2
  Product4/1 -> y_r/1
  Product3/1 -> v_r/1
  Product2/1 -> v_d_r/1
  eta_hat/1 -> Selector/1
  Selector/1 -> Integrator1/3
  rst/1 -> Integrator1/2
  Integrator1/1 -> Product4/1, Product1/3
  Product1/1 -> Sum/2
  Sum/1 -> Sum1/1
  Integrator/1 -> Saturation/1
  Product/1 -> Gain/1
  zeta/1 -> Product/3
  w_d/1 -> Product1/1, Product1/2, Product/2
  Saturation/1 -> Integrator1/1, Product/1, Product3/1
  uf/1 -> Sum/1
  Gain/1 -> Sum1/2
  Sum1/1 -> Integrator/1, Product2/1

== system Controller_CS3/Control law/Reference filter/Subsystem2 ==
  eta_hat : Inport
  rst : Inport  Port=2
  uf : Inport  Port=3
  zeta : Inport  Port=4
  w_d : Inport  Port=5
  Gain : Gain  Gain=2
  Integrator : Integrator  ExternalReset=rising
  Integrator1 : Integrator  ExternalReset=either  InitialConditionSource=external
  Product : Product  Inputs=3
  Product1 : Product  Inputs=3
  Product2 : Product
  Product3 : Product
  Product4 : Product
  Saturation : Saturate  UpperLimit=0.05  LowerLimit=-0.05
  Selector : Selector  InputPortWidth=3  Indices=[1]
  Sum : Sum  Inputs=|+-
  Sum1 : Sum  Inputs=|+-
  rst{1..4} (4 alike) : InportShadow  Port=2
  x_r : Outport
  u_r : Outport  Port=2
  u_d_r : Outport  Port=3
  wires:
  Sum1/1 -> Product2/1, Integrator/1
  Gain/1 -> Sum1/2
  uf/1 -> Sum/1
  Saturation/1 -> Product3/1, Product/1, Integrator1/1
  w_d/1 -> Product/2, Product1/2, Product1/1
  zeta/1 -> Product/3
  Product/1 -> Gain/1
  Integrator/1 -> Saturation/1
  Sum/1 -> Sum1/1
  Product1/1 -> Sum/2
  Integrator1/1 -> Product1/3, Product4/1
  rst/1 -> Integrator1/2
  Selector/1 -> Integrator1/3
  eta_hat/1 -> Selector/1
  Product2/1 -> u_d_r/1
  Product3/1 -> u_r/1
  Product4/1 -> x_r/1
  rst1/1 -> Product2/2
  rst2/1 -> Product3/2
  rst3/1 -> Product4/2
  rst4/1 -> Integrator/2

== system Controller_CS3/Control law/Reference filter/Subsystem3 ==
  eta_hat : Inport
  rst : Inport  Port=2
  uf : Inport  Port=3
  zeta : Inport  Port=4
  w_d : Inport  Port=5
  Gain : Gain  Gain=2
  Integrator : Integrator  ExternalReset=rising
  Integrator1 : Integrator  ExternalReset=either  InitialConditionSource=external
  Product : Product  Inputs=3
  Product1 : Product  Inputs=3
  Product2 : Product
  Product3 : Product
  Product4 : Product
  Saturation : Saturate  UpperLimit=5*pi/180  LowerLimit=-5*pi/180
  Selector : Selector  InputPortWidth=3  Indices=3
  Sum : Sum  Inputs=|+-
  Sum1 : Sum  Inputs=|+-
  rst{1..4} (4 alike) : InportShadow  Port=2
  psi_r : Outport
  r_r : Outport  Port=2
  r_d_r : Outport  Port=3
  wires:
  Sum1/1 -> Product2/1, Integrator/1
  Gain/1 -> Sum1/2
  uf/1 -> Sum/1
  Saturation/1 -> Product3/1, Product/1, Integrator1/1
  w_d/1 -> Product/2, Product1/2, Product1/1
  zeta/1 -> Product/3
  Product/1 -> Gain/1
  Integrator/1 -> Saturation/1
  Sum/1 -> Sum1/1
  Product1/1 -> Sum/2
  Integrator1/1 -> Product1/3, Product4/1
  rst/1 -> Integrator1/2
  Selector/1 -> Integrator1/3
  eta_hat/1 -> Selector/1
  Product2/1 -> r_d_r/1
  Product3/1 -> r_r/1
  Product4/1 -> psi_r/1
  rst1/1 -> Product2/2
  rst2/1 -> Product3/2
  rst3/1 -> Product4/2
  rst4/1 -> Integrator/2

== system Controller_CS3/Control law/Tau PD-control/GNC: "Transposed rotation matrix yaw: RTz_psi" ==
  note: GNC: "Transposed
      | rotation matrix yaw"
  psi : Inport
  nu : Inport  Port=2  PortDimensions=3
  Fcn : Fcn  Expr=cos(u(1))*u(2)+sin(u(1))*u(3)
  Fcn1 : Fcn  Expr=-sin(u(1))*u(2)+cos(u(1))*u(3)
  Fcn2 : Fcn  Expr=u(4)
  Mux2 : Mux  Inputs=2
  Mux3 : Mux  Inputs=3
  R_T*nu : Outport
  wires:
  Mux2/1 -> Fcn1/1, Fcn/1, Fcn2/1
  Fcn/1 -> Mux3/1  "x_dot"
  Fcn1/1 -> Mux3/2  "y_dot"
  Fcn2/1 -> Mux3/3  "psi_dot"
  Mux3/1 -> R_T*nu/1  "eta_dot"
  psi/1 -> Mux2/1
  nu/1 -> Mux2/2

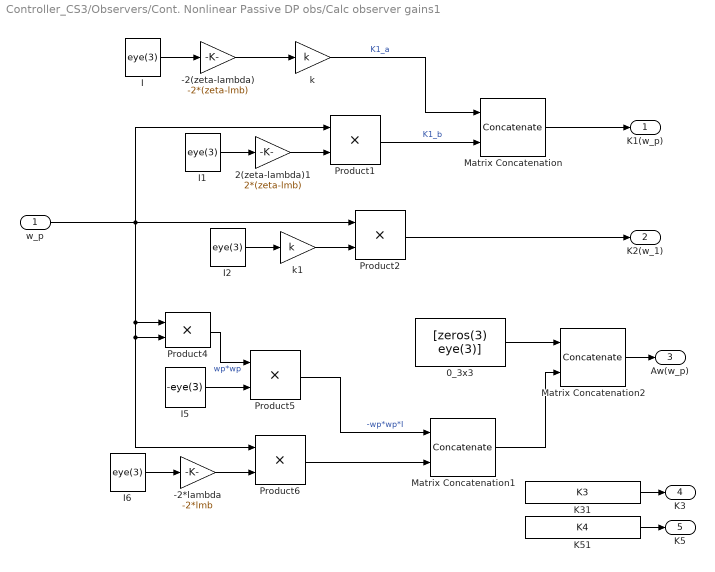
== system Controller_CS3/Observers/Cont. Nonlinear Passive DP obs/Calc observer gains1 ==
  w_p : Inport
  -2(zeta-lambda) : Gain  Gain=-2*(zeta-lmb)  SaturateOnIntegerOverflow=on  OutDataTypeStr=Inherit: Same as input  ParamDataTypeStr=Inherit: Same as input
  -2*lambda : Gain  Gain=-2*lmb  SaturateOnIntegerOverflow=on  OutDataTypeStr=Inherit: Same as input  ParamDataTypeStr=Inherit: Same as input
  0_3x3 : Constant  Value=[zeros(3) eye(3)]
  2(zeta-lambda)1 : Gain  Gain=2*(zeta-lmb)  SaturateOnIntegerOverflow=on  OutDataTypeStr=Inherit: Same as input  ParamDataTypeStr=Inherit: Same as input
  I{,1..2,6} (4 alike) : Constant  Value=eye(3)
  I5 : Constant  Value=-eye(3)
  K31 : Constant  Value=K3
  K51 : Constant  Value=K4
  Matrix Concatenation : Concatenate  Mode=Multidimensional array
  Matrix Concatenation1 : Concatenate  Mode=Multidimensional array  ConcatenateDimension=2
  Matrix Concatenation2 : Concatenate  Mode=Multidimensional array
  Product{1..2,4..6} (5 alike) : Product  SaturateOnIntegerOverflow=on  OutDataTypeStr=Inherit: Same as first input
  k : Gain  Gain=k  SaturateOnIntegerOverflow=on  OutDataTypeStr=Inherit: Same as input  ParamDataTypeStr=Inherit: Same as input
  k1 : Gain  Gain=k  SaturateOnIntegerOverflow=on  OutDataTypeStr=Inherit: Same as input  ParamDataTypeStr=Inherit: Same as input
  K1(w_p) : Outport
  K2(w_1) : Outport  Port=2
  Aw(w_p) : Outport  Port=3
  K3 : Outport  Port=4
  K5 : Outport  Port=5
  wires:
  K51/1 -> K5/1
  K31/1 -> K3/1
  Matrix Concatenation2/1 -> Aw(w_p)/1
  0_3x3/1 -> Matrix Concatenation2/1
  Matrix Concatenation1/1 -> Matrix Concatenation2/2
  Product6/1 -> Matrix Concatenation1/2
  -2*lambda/1 -> Product6/2
  I6/1 -> -2*lambda/1
  Product5/1 -> Matrix Concatenation1/1  "-wp*wp*I"
  I5/1 -> Product5/2
  Product4/1 -> Product5/1  "wp*wp"
  k/1 -> Matrix Concatenation/1  "K1_a"
  k1/1 -> Product2/2
  Product2/1 -> K2(w_1)/1
  I2/1 -> k1/1
  Product1/1 -> Matrix Concatenation/2  "K1_b"
  2(zeta-lambda)1/1 -> Product1/2
  I1/1 -> 2(zeta-lambda)1/1
  -2(zeta-lambda)/1 -> k/1
  I/1 -> -2(zeta-lambda)/1
  w_p/1 -> Product6/1, Product4/2, Product4/1, Product2/1, Product1/1
  Matrix Concatenation/1 -> K1(w_p)/1

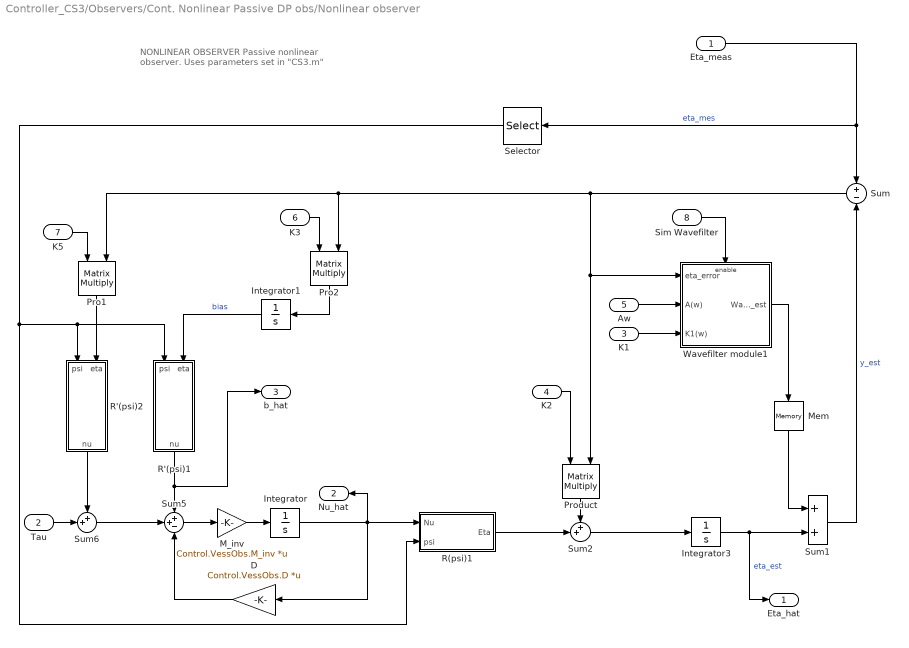
== system Controller_CS3/Observers/Cont. Nonlinear Passive DP obs/Nonlinear observer ==
  note: NONLINEAR OBSERVER
      | Passive nonlinear observer. Uses parameters
      | set in "CS3.m"
  Eta_meas : Inport
  Tau : Inport  Port=2
  K1 : Inport  Port=3
  K2 : Inport  Port=4
  Aw : Inport  Port=5
  K3 : Inport  Port=6
  K5 : Inport  Port=7
  Sim Wavefilter : Inport  Port=8
  D : Gain  Gain=Control.VessObs.D  Multiplication=Matrix(K*u)  SaturateOnIntegerOverflow=on  OutDataTypeStr=Inherit: Same as input  ParamDataTypeStr=Inherit: Same as input
  Integrator : Integrator
  Integrator1 : Integrator
  Integrator3 : Integrator
  M_inv : Gain  Gain=Control.VessObs.M_inv  Multiplication=Matrix(K*u)  SaturateOnIntegerOverflow=on  OutDataTypeStr=Inherit: Same as input  ParamDataTypeStr=Inherit: Same as input
  Mem : Memory
  Pro1 : Product  Multiplication=Matrix(*)  SaturateOnIntegerOverflow=on  OutDataTypeStr=Inherit: Same as first input
  Pro2 : Product  Multiplication=Matrix(*)  SaturateOnIntegerOverflow=on  OutDataTypeStr=Inherit: Same as first input
  Product : Product  Multiplication=Matrix(*)  SaturateOnIntegerOverflow=on  OutDataTypeStr=Inherit: Same as first input
  R'(psi)1 : Subsystem
  R'(psi)2 : Subsystem
  R(psi)1 : Subsystem
  Selector : Selector  InputPortWidth=3  Indices=3
  Sum : Sum  Inputs=+-  SaturateOnIntegerOverflow=on
  Sum1 : Sum  SaturateOnIntegerOverflow=on
  Sum2 : Sum  Inputs=++|  SaturateOnIntegerOverflow=on
  Sum5 : Sum  Inputs=++-  SaturateOnIntegerOverflow=on
  Sum6 : Sum  Inputs=++|  SaturateOnIntegerOverflow=on
  Wavefilter module1 : Subsystem
  Eta_hat : Outport  InitialOutput=0
  Nu_hat : Outport  Port=2  InitialOutput=0
  b_hat : Outport  Port=3  InitialOutput=0
  wires:
  Pro2/1 -> Integrator1/1
  Sim Wavefilter/1 -> Wavefilter module1/Enable
  Sum1/1 -> Sum/2  "y_est"
  Mem/1 -> Sum1/1
  Selector/1 -> R(psi)1/2(psi), R'(psi)1/1(psi), R'(psi)2/1(psi)
  K5/1 -> Pro1/1
  K3/1 -> Pro2/1
  K2/1 -> Product/1
  Product/1 -> Sum2/1
  K1/1 -> Wavefilter module1/3(K1(w))
  Eta_meas/1 -> Selector/1, Sum/1  "eta_mes"
  M_inv/1 -> Integrator/1
  Integrator/1 -> Nu_hat/1, D/1, R(psi)1/1(Nu)
  Pro1/1 -> R'(psi)2/2(eta)
  Tau/1 -> Sum6/2
  R(psi)1/1(Eta) -> Sum2/2
  R'(psi)1/1(nu) -> b_hat/1, Sum5/1
  R'(psi)2/1(nu) -> Sum6/1
  Wavefilter module1/1(Wave_est) -> Mem/1
  Sum6/1 -> Sum5/2
  D/1 -> Sum5/3
  Sum5/1 -> M_inv/1
  Integrator1/1 -> R'(psi)1/2(eta)  "bias"
  Sum2/1 -> Integrator3/1
  Sum/1 -> Pro2/2, Pro1/2, Product/2, Wavefilter module1/1(eta_error)
  Integrator3/1 -> Eta_hat/1, Sum1/2  "eta_est"
  Aw/1 -> Wavefilter module1/2(A(w))

== system Controller_CS3/Observers/Hybrid Nonlinear Passive DP obs/Cx block ==
  x : Inport
  wave_filter : Inport  Port=2
  Product : Product
  Selector : Selector  InputPortWidth=15  Indices=[7 8 9]
  Selector1 : Selector  InputPortWidth=15  Indices=[4 5 6]
  Sum : Sum  Inputs=|++
  Cx : Outport
  wires:
  x/1 -> Selector1/1, Selector/1
  Selector1/1 -> Product/2
  wave_filter/1 -> Product/1
  Product/1 -> Sum/1
  Selector/1 -> Sum/2
  Sum/1 -> Cx/1

== system Controller_CS3/Observers/Hybrid Nonlinear Passive DP obs/Error filter ==
  e : Inport
  gs : Inport  Port=2
  Demux : Demux  Outputs=3
  Demux1 : Demux  Outputs=3
  Mux : Mux  Inputs=3
  Mux1 : Mux  Inputs=2
  Scope : Scope
  Subsystem : Subsystem
  Subsystem1 : Subsystem
  Subsystem2 : Subsystem
  e_f : Outport  PortDimensions=3
  wires:
  Mux/1 -> e_f/1
  Subsystem/1(Out1) -> Mux1/2, Mux/1
  Subsystem1/1(Out1) -> Mux/2
  Subsystem2/1(Out1) -> Mux/3
  e/1 -> Demux/1
  Demux/1 -> Mux1/1, Subsystem/1(In1)
  Demux/2 -> Subsystem1/1(In1)
  Demux/3 -> Subsystem2/1(In1)
  gs/1 -> Demux1/1
  Demux1/1 -> Subsystem/2(gs)
  Demux1/2 -> Subsystem1/2(gs)
  Demux1/3 -> Subsystem2/2(gs)
  Mux1/1 -> Scope/1

== system Controller_CS3/Observers/Hybrid Nonlinear Passive DP obs/Integrator system ==
  f : Inport
  g : Inport  Port=2
  D : Inport  Port=3
  CT dynamics : Subsystem
  Demux : Demux  Outputs=3
  Demux1 : Demux  Outputs=3
  ICx : InitialCondition  Value=zeros(15,1)
  ICx0 : InitialCondition  Value=[0; 0; zeros(15,1)]
  Integrator : Integrator  ExternalReset=level hold  InitialConditionSource=external  ShowStatePort=on  ZeroCross=off
  Update logic : Subsystem
  x : Outport
  t : Outport  Port=2
  j : Outport  Port=3
  x- : Outport  Port=4  PortDimensions=15
  wires:
  Integrator/State -> Demux1/1
  CT dynamics/1(dot) -> Integrator/1
  Demux/2 -> j/1
  ICx/1 -> x/1
  Demux/1 -> t/1
  D/1 -> Integrator/2
  Integrator/1 -> Demux/1
  Demux/3 -> ICx/1
  ICx0/1 -> Integrator/3
  Update logic/1(update law) -> ICx0/1
  g/1 -> Update logic/1(g(x-,u))
  f/1 -> CT dynamics/1(f(x,u))
  Demux1/1 -> Update logic/3(t-)
  Demux1/2 -> Update logic/2(j-)
  Demux1/3 -> x-/1

== system Controller_CS3/Observers/Hybrid Nonlinear Passive DP obs/Jump map ==
  x : Inport
  y : Inport  Port=2
  w_p : Inport  Port=3
  e : Inport  Port=4
  g_max : Inport  Port=5
  gs : Inport  Port=6
  wave_filter : Inport  Port=7
  Enable : EnablePort
  Calc observer gains1 : Subsystem  mask{lmb=Control.VessObs.lmb{2}, k=Control.VessObs.k{2}, zeta=Control.VessObs.damp{2}, K3=Control.VessObs.K3{2}, K4=Control.VessObs.K4{2}}
      mask prompts: lmb "Control.VessObs.lmb{i}=lmb"; k "Control.VessObs.k{i}=k"; zeta "Control.VessObs.damp{i}=zeta"; K3 "Control.VessObs.K3{1}=K3"; K4 "Control.VessObs.K4{1}=K4"
  D : Constant  Value=Control.VessObs.D
  M_inv : Constant  Value=Control.VessObs.M_inv
  jump map g : MATLAB Function  TreatAsAtomicUnit=on
  g : Outport
  wires:
  x/1 -> jump map g/1(x)
  D/1 -> jump map g/9(D)
  M_inv/1 -> jump map g/8(M_inv)
  Calc observer gains1/5(K5) -> jump map g/7(K5)
  Calc observer gains1/1(K1(w_p)) -> jump map g/3(K1)
  Calc observer gains1/4(K3) -> jump map g/6(K3)
  Calc observer gains1/2(K2(w_1)) -> jump map g/4(K2)
  Calc observer gains1/3(Aw(w_p)) -> jump map g/5(Aw)
  jump map g/1(x_plus) -> g/1
  wave_filter/1 -> jump map g/13(wave_filter_onoff)
  y/1 -> jump map g/2(y)
  w_p/1 -> Calc observer gains1/1(w_p)
  g_max/1 -> jump map g/11(g_max)
  e/1 -> jump map g/10(e)
  gs/1 -> jump map g/12(gs)

== system Controller_CS3/Observers/Hybrid Nonlinear Passive DP obs/R'(psi)1 ==
  psi : Inport
  eta : Inport  Port=2
  Demux : Demux  Outputs=3
  Mux : Mux  Inputs=3
  Mux1 : Mux  Inputs=3
  Row1 : Fcn  Expr=cos(u(3))*u(1)+sin(u(3))*u(2)
  Row2 : Fcn  Expr=-sin(u(3))*u(1)+cos(u(3))*u(2)
  nu : Outport
  wires:
  Row1/1 -> Mux1/1
  Row2/1 -> Mux1/2
  Mux1/1 -> nu/1
  Mux/1 -> Row2/1, Row1/1
  eta/1 -> Demux/1
  psi/1 -> Mux/3
  Demux/1 -> Mux/1
  Demux/2 -> Mux/2
  Demux/3 -> Mux1/3

== system Controller_CS3/Observers/Hybrid Nonlinear Passive DP obs/flow map ==
  x : Inport
  y : Inport  Port=2
  tau : Inport  Port=3
  w_p : Inport  Port=4
  wave_filter : Inport  Port=5
  Calc observer gains1 : Subsystem  mask{lmb=Control.VessObs.lmb{2}, k=Control.VessObs.k{2}, zeta=Control.VessObs.damp{2}, K3=Control.VessObs.K3{2}, K4=Control.VessObs.K4{2}}
      mask prompts: lmb "Control.VessObs.lmb{i}=lmb"; k "Control.VessObs.k{i}=k"; zeta "Control.VessObs.damp{i}=zeta"; K3 "Control.VessObs.K3{1}=K3"; K4 "Control.VessObs.K4{1}=K4"
  D : Constant  Value=Control.VessObs.D
  M_inv : Constant  Value=Control.VessObs.M_inv
  flow map f : MATLAB Function  TreatAsAtomicUnit=on
  f : Outport
  wires:
  w_p/1 -> Calc observer gains1/1(w_p)
  y/1 -> flow map f/2(y)
  tau/1 -> flow map f/3(tau)
  flow map f/1(xdot) -> f/1
  Calc observer gains1/3(Aw(w_p)) -> flow map f/6(Aw)
  Calc observer gains1/2(K2(w_1)) -> flow map f/5(K2)
  Calc observer gains1/4(K3) -> flow map f/7(K3)
  Calc observer gains1/1(K1(w_p)) -> flow map f/4(K1)
  Calc observer gains1/5(K5) -> flow map f/8(K5)
  M_inv/1 -> flow map f/9(M_inv)
  D/1 -> flow map f/10(D)
  x/1 -> flow map f/1(x)
  wave_filter/1 -> flow map f/11(wave_filter_onoff)

== system Controller_CS3/Observers/Cont. Nonlinear Passive DP obs/Nonlinear observer/R'(psi)1 ==
  psi : Inport
  eta : Inport  Port=2
  Demux : Demux  Outputs=3
  Mux : Mux  Inputs=3
  Mux1 : Mux  Inputs=3
  Row1 : Fcn  Expr=cos(u(3))*u(1)+sin(u(3))*u(2)
  Row2 : Fcn  Expr=-sin(u(3))*u(1)+cos(u(3))*u(2)
  nu : Outport
  wires:
  Row1/1 -> Mux1/1
  Row2/1 -> Mux1/2
  Mux1/1 -> nu/1
  Mux/1 -> Row2/1, Row1/1
  eta/1 -> Demux/1
  psi/1 -> Mux/3
  Demux/1 -> Mux/1
  Demux/2 -> Mux/2
  Demux/3 -> Mux1/3

== system Controller_CS3/Observers/Cont. Nonlinear Passive DP obs/Nonlinear observer/R'(psi)2 ==
  psi : Inport
  eta : Inport  Port=2
  Demux : Demux  Outputs=3
  Mux : Mux  Inputs=3
  Mux1 : Mux  Inputs=3
  Row1 : Fcn  Expr=cos(u(3))*u(1)+sin(u(3))*u(2)
  Row2 : Fcn  Expr=-sin(u(3))*u(1)+cos(u(3))*u(2)
  nu : Outport
  wires:
  Demux/3 -> Mux1/3
  Demux/2 -> Mux/2
  Demux/1 -> Mux/1
  psi/1 -> Mux/3
  eta/1 -> Demux/1
  Mux/1 -> Row1/1, Row2/1
  Mux1/1 -> nu/1
  Row2/1 -> Mux1/2
  Row1/1 -> Mux1/1

== system Controller_CS3/Observers/Cont. Nonlinear Passive DP obs/Nonlinear observer/R(psi)1 ==
  Nu : Inport
  psi : Inport  Port=2
  Demux : Demux  Outputs=3
  Mux : Mux  Inputs=3
  Mux1 : Mux  Inputs=3
  Row1 : Fcn  Expr=cos(u(3))*u(1)-sin(u(3))*u(2)
  Row2 : Fcn  Expr=sin(u(3))*u(1)+cos(u(3))*u(2)
  Eta : Outport
  wires:
  Demux/3 -> Mux1/3
  Nu/1 -> Demux/1
  psi/1 -> Mux/3
  Demux/1 -> Mux/1
  Demux/2 -> Mux/2
  Mux/1 -> Row2/1, Row1/1
  Mux1/1 -> Eta/1
  Row2/1 -> Mux1/2
  Row1/1 -> Mux1/1
